simulink model "PRO_TestHarness"  (Simulink 8.6)
settings: Solver=ode45  StartTime=0.0  StopTime=10.0  RelTol=1e-3
PreLoadFcn:
  | addpath('./Workspace/')
  | load('./Workspace/EnvVar.mat')
  | if exist('tl_preloadfcn','file'), tl_preloadfcn(gcs,402); end
PostLoadFcn:
  | if exist('tl_postloadfcn','file'), tl_postloadfcn(gcs,402); end
InitFcn:
  | if exist('tlds_init','file'), tlds_init(gcs); end
StartFcn:
  | if exist('tlds_start','file'), tlds_start(gcs); end
StopFcn:
  | if exist('tlds_stop','file'), tlds_stop(gcs); end
undefined symbols (not defined in the file or in its folder): ddv, sigbuilder_block, Ts
libraries: tllib x19, simulink x2
(part 4 of 5)

== system PRO_TestHarness/PRO_AC_ProductionCycles/Subsystem/PRO_AC_ProductionCycles/PRO_AC_ProductionCycles/PRO_runProductionCycles/PRO enabled/FctCommonPROManageInputs/FctCommonEvaluatePreConditions ==
  b8SystemContextInhibition : Inport  OutDataTypeStr=uint8  PortDimensions=1
  b8SystemContextAbortion : Inport  Port=2  OutDataTypeStr=uint8  PortDimensions=1
  bNoInhibitionByUVDuringTensioning : Inport  Port=3  OutDataTypeStr=boolean
  u8OverVoltageEventStatus : Inport  Port=4
  Bitwise Operator : tllib/Bitwise Operator  logicop=AND  UseBitMask=off  NumInputPorts=2  BitMask=bin2dec('11011001')  BitMaskRealWorld=Stored Integer  data={'date',735742.74357686343}
  Constant2 : Constant  Value=ddv('BFD/KU8_CONTEXT_STATUS_ON')  OutDataTypeStr=uint8  mask(TL_Constant){data={'output',{'variable','BFD/KU8_CONTEXT_STATUS_ON'},'date',735893.58242878469}}
      settings: DeleteFcn=if exist('delete_tlblock','file')==2,delete_tlblock(gcbh);end  NameChangeFcn=if exist('rename_tlblock','file')==2,rename_tlblock(gcbh);end  OpenFcn=if exist('tl_open_blockdlg','file')==2,tl_open_blockdlg(gcbh);else,open_system(gcbh,'parameter');end
      mask Help: eval(['if exist(''tl_online_help'',''file'') == 2, tl_online_help(''Topic'',''TL_Constant''),else, web([''jar:file:///'',matlabroot,''/help/toolbox/simulink/help.jar!/slref/' lower(get_param(gcbh,'Blocktype')) '.html''], ''-helpbrowser''),end'])
      mask Display: plot([-0.05, 1.05, NaN, -0.05, 1.05],[.01, .01, NaN, .99, .99])
  Constant3 : Constant  Value=ddv('BFD/KU8_ZERO')  OutDataTypeStr=uint8  mask(TL_Constant){data={'output',{'variable','BFD/KU8_ZERO'},'date',735742.74390618061}}
      settings: DeleteFcn=if exist('delete_tlblock','file')==2,delete_tlblock(gcbh);end  NameChangeFcn=if exist('rename_tlblock','file')==2,rename_tlblock(gcbh);end  OpenFcn=if exist('tl_open_blockdlg','file')==2,tl_open_blockdlg(gcbh);else,open_system(gcbh,'parameter');end
      mask Help: eval(['if exist(''tl_online_help'',''file'') == 2, tl_online_help(''Topic'',''TL_Constant''),else, web([''jar:file:///'',matlabroot,''/help/toolbox/simulink/help.jar!/slref/' lower(get_param(gcbh,'Blocktype')) '.html''], ''-helpbrowser''),end'])
      mask Display: plot([-0.05, 1.05, NaN, -0.05, 1.05],[.01, .01, NaN, .99, .99])
  Constant4 : Constant  Value=ddv('BFD/KU8_CONTEXT_STATUS_ON')  OutDataTypeStr=uint8  mask(TL_Constant){data={'output',{'variable','BFD/KU8_CONTEXT_STATUS_ON'},'date',735893.58242917829}}
      settings: DeleteFcn=if exist('delete_tlblock','file')==2,delete_tlblock(gcbh);end  NameChangeFcn=if exist('rename_tlblock','file')==2,rename_tlblock(gcbh);end  OpenFcn=if exist('tl_open_blockdlg','file')==2,tl_open_blockdlg(gcbh);else,open_system(gcbh,'parameter');end
      mask Help: eval(['if exist(''tl_online_help'',''file'') == 2, tl_online_help(''Topic'',''TL_Constant''),else, web([''jar:file:///'',matlabroot,''/help/toolbox/simulink/help.jar!/slref/' lower(get_param(gcbh,'Blocktype')) '.html''], ''-helpbrowser''),end'])
      mask Display: plot([-0.05, 1.05, NaN, -0.05, 1.05],[.01, .01, NaN, .99, .99])
  Constant5 : Constant  Value=ddv('RTE_DEFINES/DEM_UDS_STATUS_TF')  OutDataTypeStr=uint8  mask(TL_Constant){data={'output',{'variable','RTE_DEFINES/DEM_UDS_STATUS_TF'},'date',736811.33803680551}}
      settings: DeleteFcn=if exist('delete_tlblock','file')==2,delete_tlblock(gcbh);end  NameChangeFcn=if exist('rename_tlblock','file')==2,rename_tlblock(gcbh);end  OpenFcn=if exist('tl_open_blockdlg','file')==2,tl_open_blockdlg(gcbh);else,open_system(gcbh,'parameter');end
      mask Help: eval(['if exist(''tl_online_help'',''file'') == 2, tl_online_help(''Topic'',''TL_Constant''),else, web([''jar:file:///'',matlabroot,''/help/toolbox/simulink/help.jar!/slref/' lower(get_param(gcbh,'Blocktype')) '.html''], ''-helpbrowser''),end'])
      mask Display: plot([-0.05, 1.05, NaN, -0.05, 1.05],[.01, .01, NaN, .99, .99])
  Function : tllib/Function  data={'stepfunctionname','EvaluatePreConditionsForAllPRO','stepfunctionclass','STATIC_FCN_ASR4','codecomment',['This function is in charge of' char(10) 'providing the following outputs:' char(10) '' char(10) '- the common PRO preconditions flag' char(10) '' char(10) 'according to the inputs:' char(10) '' char(10) '- inhibition context' char(10) '- abortion context'],'module','PRO_AC_ProductionCycles','date',736463.55392600689}  displayString=FUNCTION
  Relational Operator3 : RelationalOperator  Operator=~=  OutDataTypeStr=boolean  mask(TL_RelationalOperator){data={'date',735893.57161760412}}
      settings: DeleteFcn=if exist('delete_tlblock','file')==2,delete_tlblock(gcbh);end  NameChangeFcn=if exist('rename_tlblock','file')==2,rename_tlblock(gcbh);end  OpenFcn=if exist('tl_open_blockdlg','file')==2,tl_open_blockdlg(gcbh);else,open_system(gcbh,'parameter');end
      mask Help: eval(['if exist(''tl_online_help'',''file'') == 2, tl_online_help(''Topic'',''TL_RelationalOperator''),else, web([''jar:file:///'',matlabroot,''/help/toolbox/simulink/help.jar!/slref/' lower(get_param(gcbh,'Blocktype')) '.html''], ''-helpbrowser''),end'])
      mask Display: plot([-0.05, 1.05, NaN, -0.05, 1.05],[.01, .01, NaN, .99, .99])
  Relational Operator4 : RelationalOperator  Operator=~=  OutDataTypeStr=boolean  mask(TL_RelationalOperator){data={'date',735893.57182078704}}
      settings: DeleteFcn=if exist('delete_tlblock','file')==2,delete_tlblock(gcbh);end  NameChangeFcn=if exist('rename_tlblock','file')==2,rename_tlblock(gcbh);end  OpenFcn=if exist('tl_open_blockdlg','file')==2,tl_open_blockdlg(gcbh);else,open_system(gcbh,'parameter');end
      mask Help: eval(['if exist(''tl_online_help'',''file'') == 2, tl_online_help(''Topic'',''TL_RelationalOperator''),else, web([''jar:file:///'',matlabroot,''/help/toolbox/simulink/help.jar!/slref/' lower(get_param(gcbh,'Blocktype')) '.html''], ''-helpbrowser''),end'])
      mask Display: plot([-0.05, 1.05, NaN, -0.05, 1.05],[.01, .01, NaN, .99, .99])
  bOVONotQualified : RelationalOperator  Operator===  OutDataTypeStr=boolean  mask(TL_RelationalOperator){data={'output',{'name','$B'},'date',735987.61379924766}}
      settings: DeleteFcn=if exist('delete_tlblock','file')==2,delete_tlblock(gcbh);end  NameChangeFcn=if exist('rename_tlblock','file')==2,rename_tlblock(gcbh);end  OpenFcn=if exist('tl_open_blockdlg','file')==2,tl_open_blockdlg(gcbh);else,open_system(gcbh,'parameter');end
      mask Help: eval(['if exist(''tl_online_help'',''file'') == 2, tl_online_help(''Topic'',''TL_RelationalOperator''),else, web([''jar:file:///'',matlabroot,''/help/toolbox/simulink/help.jar!/slref/' lower(get_param(gcbh,'Blocktype')) '.html''], ''-helpbrowser''),end'])
      mask Display: plot([-0.05, 1.05, NaN, -0.05, 1.05],[.01, .01, NaN, .99, .99])
  bPreConditionsFlag_PRO : Logic  Inputs=4  AllPortsSameDT=off  OutDataTypeStr=boolean  mask(TL_LogicalOperator){data={'output',{'name','$B'},'date',735986.42247924767}}
      settings: DeleteFcn=if exist('delete_tlblock','file')==2,delete_tlblock(gcbh);end  NameChangeFcn=if exist('rename_tlblock','file')==2,rename_tlblock(gcbh);end  OpenFcn=if exist('tl_open_blockdlg','file')==2,tl_open_blockdlg(gcbh);else,open_system(gcbh,'parameter');end
      mask Help: eval(['if exist(''tl_online_help'',''file'') == 2, tl_online_help(''Topic'',''TL_LogicalOperator''),else, web([''jar:file:///'',matlabroot,''/help/toolbox/simulink/help.jar!/slref/' lower(get_param(gcbh,'Blocktype')) '.html''], ''-helpbrowser''),end'])
      mask Display: plot([-0.05, 1.05, NaN, -0.05, 1.05],[.01, .01, NaN, .99, .99])
  bPreConditionsFlagT_out : Outport  InitialOutput=[0]
  wires:
  b8SystemContextInhibition/1 -> Relational Operator3/1
  Constant2/1 -> Relational Operator3/2
  Constant4/1 -> Relational Operator4/2
  b8SystemContextAbortion/1 -> Relational Operator4/1
  Relational Operator4/1 -> bPreConditionsFlag_PRO/2
  Relational Operator3/1 -> bPreConditionsFlag_PRO/1
  bPreConditionsFlag_PRO/1 -> bPreConditionsFlagT_out/1
  bNoInhibitionByUVDuringTensioning/1 -> bPreConditionsFlag_PRO/3
  bOVONotQualified/1 -> bPreConditionsFlag_PRO/4
  Constant5/1 -> Bitwise Operator/2
  Bitwise Operator/1 -> bOVONotQualified/1
  Constant3/1 -> bOVONotQualified/2
  u8OverVoltageEventStatus/1 -> Bitwise Operator/1

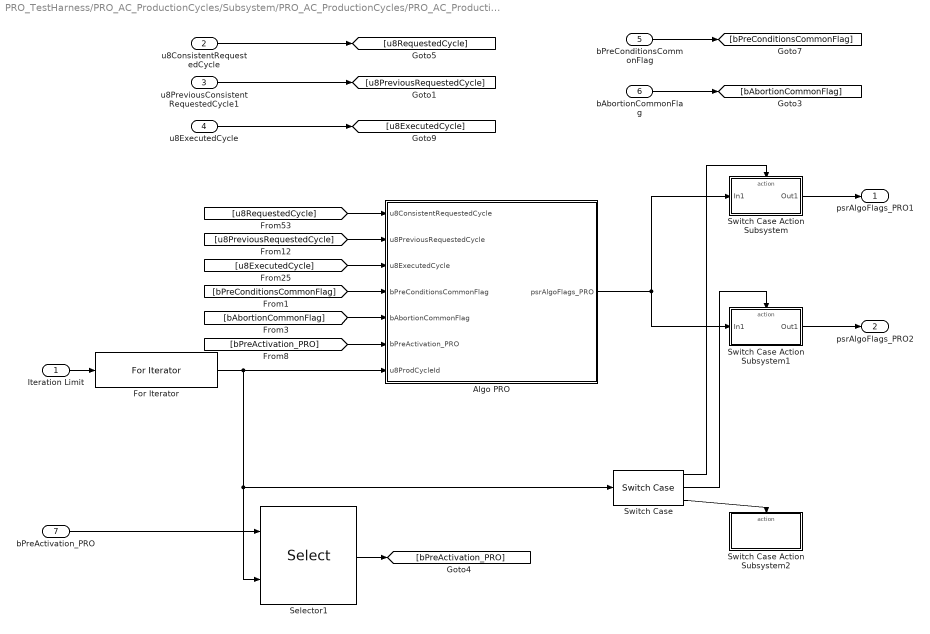
== system PRO_TestHarness/PRO_AC_ProductionCycles/Subsystem/PRO_AC_ProductionCycles/PRO_AC_ProductionCycles/PRO_runProductionCycles/PRO enabled/FctTrigAbortCycle_AllPRO/For Iterator Subsystem ==
  Iteration Limit : Inport
  u8ConsistentRequestedCycle : Inport  Port=2  OutDataTypeStr=uint8  PortDimensions=1
  u8PreviousConsistentRequestedCycle1 : Inport  Port=3  OutDataTypeStr=uint8  PortDimensions=1
  u8ExecutedCycle : Inport  Port=4  PortDimensions=1
  bPreConditionsCommonFlag : Inport  Port=5
  bAbortionCommonFlag : Inport  Port=6  PortDimensions=1
  bPreActivation_PRO : Inport  Port=7
  Algo PRO : Subsystem
  For Iterator : ForIterator  IterationSource=external  IndexMode=Zero-based  IterationVariableDataType=int8
  Selector1 : Selector  IndexMode=Zero-based  InputPortWidth=2  IndexOptions=Index vector (port)  Indices=[1 3]  OutputSizes=1
  Switch Case : SwitchCase  CaseConditions={0,1}
  Switch Case Action Subsystem : Subsystem  TreatAsAtomicUnit=on
  Switch Case Action Subsystem1 : Subsystem  TreatAsAtomicUnit=on
  Switch Case Action Subsystem2 : Subsystem  TreatAsAtomicUnit=on
  psrAlgoFlags_PRO1 : Outport
  psrAlgoFlags_PRO2 : Outport  Port=2
  wires:
  Algo PRO/1(psrAlgoFlags_PRO) -> Switch Case Action Subsystem1/1(In1), Switch Case Action Subsystem/1(In1)
  Iteration Limit/1 -> For Iterator/1
  u8ExecutedCycle/1 -> [u8ExecutedCycle]
  bAbortionCommonFlag/1 -> [bAbortionCommonFlag]
  bPreConditionsCommonFlag/1 -> [bPreConditionsCommonFlag]
  u8ConsistentRequestedCycle/1 -> [u8RequestedCycle]
  bPreActivation_PRO/1 -> Selector1/1
  u8PreviousConsistentRequestedCycle1/1 -> [u8PreviousRequestedCycle]
  For Iterator/1 -> Selector1/2, Switch Case/1, Algo PRO/7(u8ProdCycleId)
  [bPreConditionsCommonFlag] -> Algo PRO/4(bPreConditionsCommonFlag)
  [u8RequestedCycle] -> Algo PRO/1(u8ConsistentRequestedCycle)
  [bPreActivation_PRO] -> Algo PRO/6(bPreActivation_PRO)
  [bAbortionCommonFlag] -> Algo PRO/5(bAbortionCommonFlag)
  [u8PreviousRequestedCycle] -> Algo PRO/2(u8PreviousRequestedCycle)
  [u8ExecutedCycle] -> Algo PRO/3(u8ExecutedCycle)
  Switch Case/1 -> Switch Case Action Subsystem/Action
  Switch Case Action Subsystem/1(Out1) -> psrAlgoFlags_PRO1/1
  Switch Case Action Subsystem1/1(Out1) -> psrAlgoFlags_PRO2/1
  Switch Case/2 -> Switch Case Action Subsystem1/Action
  Switch Case/3 -> Switch Case Action Subsystem2/Action
  Selector1/1 -> [bPreActivation_PRO]

== system PRO_TestHarness/PRO_AC_ProductionCycles/Subsystem/PRO_AC_ProductionCycles/PRO_AC_ProductionCycles/PRO_runProductionCycles/PRO enabled/FctCommonPROManageInputs/FctCheckUnderVoltageDuringTensioningForAllPRO/For Iterator Subsystem ==
  In1 : Inport
  bPreActivationFlag_PRO : Inport  Port=2
  bPreActivationFlag_PRO_UnitDelay : Inport  Port=3
  Constant : Constant  Value=0  OutDataTypeStr=boolean  mask(TL_Constant){data={'date',736182.47245412041}}
      settings: CopyFcn=if exist('tl_reset_reviewflag') == 2, tl_reset_reviewflag(gcbh); end  DeleteFcn=if exist('delete_tlblock','file')==2,delete_tlblock(gcbh);end  NameChangeFcn=if exist('rename_tlblock','file')==2,rename_tlblock(gcbh);end  OpenFcn=if exist('tl_open_blockdlg','file')==2,tl_open_blockdlg(gcbh);else,open_system(gcbh,'parameter');end
      mask Help: eval(['if exist(''tl_online_help'',''file'') == 2, tl_online_help(''Topic'',''TL_Constant''),else, web([''jar:file:///'',matlabroot,''/help/toolbox/simulink/help.jar!/slref/' lower(get_param(gcbh,'Blocktype')) '.html''], ''-helpbrowser''),end'])
      mask Display: plot([-0.05, 1.05, NaN, -0.05, 1.05],[.01, .01, NaN, .99, .99])
  For Iterator : ForIterator  IterationSource=external  IndexMode=Zero-based  IterationVariableDataType=int8
  Selector : Selector  IndexMode=Zero-based  InputPortWidth=2  IndexOptions=Index vector (port)  Indices=[1 3]  OutputSizes=1
  Selector1 : Selector  IndexMode=Zero-based  InputPortWidth=2  IndexOptions=Index vector (port)  Indices=[1 3]  OutputSizes=1
  Switch : Switch  Criteria=u2 ~= 0  mask(TL_Switch){data={'output',{'type','Bool'},'date',736182.47204471065}}
      settings: CopyFcn=if exist('tl_reset_reviewflag') == 2, tl_reset_reviewflag(gcbh); end  DeleteFcn=if exist('delete_tlblock','file')==2,delete_tlblock(gcbh);end  NameChangeFcn=if exist('rename_tlblock','file')==2,rename_tlblock(gcbh);end  OpenFcn=if exist('tl_open_blockdlg','file')==2,tl_open_blockdlg(gcbh);else,open_system(gcbh,'parameter');end
      mask Help: eval(['if exist(''tl_online_help'',''file'') == 2, tl_online_help(''Topic'',''TL_Switch''),else, web([''jar:file:///'',matlabroot,''/help/toolbox/simulink/help.jar!/slref/' lower(get_param(gcbh,'Blocktype')) '.html''], ''-helpbrowser''),end'])
      mask Display: plot([-0.05, 1.05, NaN, -0.05, 1.05],[.01, .01, NaN, .99, .99])
  Unit Delay : UnitDelay  SampleTime=-1  mask(TL_UnitDelay){data={'output',{'type','Bool'},'state',{'name','X_bIterationMemory','type','Bool'},'date',736182.47589184029}}
      settings: CopyFcn=if exist('tl_reset_reviewflag') == 2, tl_reset_reviewflag(gcbh); end  DeleteFcn=if exist('delete_tlblock','file')==2,delete_tlblock(gcbh);end  NameChangeFcn=if exist('rename_tlblock','file')==2,rename_tlblock(gcbh);end  OpenFcn=if exist('tl_open_blockdlg','file')==2,tl_open_blockdlg(gcbh);else,open_system(gcbh,'parameter');end
      mask Help: eval(['if exist(''tl_online_help'',''file'') == 2, tl_online_help(''Topic'',''TL_UnitDelay''),else, web([''jar:file:///'',matlabroot,''/help/toolbox/simulink/help.jar!/slref/' lower(get_param(gcbh,'Blocktype')) '.html''], ''-helpbrowser''),end'])
      mask Display: plot([-0.05, 1.05, NaN, -0.05, 1.05],[.01, .01, NaN, .99, .99])
  bNewRequest : Logic  AllPortsSameDT=off  OutDataTypeStr=boolean  mask(TL_LogicalOperator){data={'output',{'name','$B'},'date',735907.68610908568}}
      settings: DeleteFcn=if exist('delete_tlblock','file')==2,delete_tlblock(gcbh);end  NameChangeFcn=if exist('rename_tlblock','file')==2,rename_tlblock(gcbh);end  OpenFcn=if exist('tl_open_blockdlg','file')==2,tl_open_blockdlg(gcbh);else,open_system(gcbh,'parameter');end
      mask Help: eval(['if exist(''tl_online_help'',''file'') == 2, tl_online_help(''Topic'',''TL_LogicalOperator''),else, web([''jar:file:///'',matlabroot,''/help/toolbox/simulink/help.jar!/slref/' lower(get_param(gcbh,'Blocktype')) '.html''], ''-helpbrowser''),end'])
      mask Display: plot([-0.05, 1.05, NaN, -0.05, 1.05],[.01, .01, NaN, .99, .99])
  bNewRequest_PRO : Logic  Operator=OR  AllPortsSameDT=off  OutDataTypeStr=boolean  mask(TL_LogicalOperator){data={'output',{'name','$B'},'date',736182.47130738432}}
      settings: DeleteFcn=if exist('delete_tlblock','file')==2,delete_tlblock(gcbh);end  NameChangeFcn=if exist('rename_tlblock','file')==2,rename_tlblock(gcbh);end  OpenFcn=if exist('tl_open_blockdlg','file')==2,tl_open_blockdlg(gcbh);else,open_system(gcbh,'parameter');end
      mask Help: eval(['if exist(''tl_online_help'',''file'') == 2, tl_online_help(''Topic'',''TL_LogicalOperator''),else, web([''jar:file:///'',matlabroot,''/help/toolbox/simulink/help.jar!/slref/' lower(get_param(gcbh,'Blocktype')) '.html''], ''-helpbrowser''),end'])
      mask Display: plot([-0.05, 1.05, NaN, -0.05, 1.05],[.01, .01, NaN, .99, .99])
  bNoPreviousPreActivation_PRO : Logic  Operator=NOT  Inputs=1  AllPortsSameDT=off  OutDataTypeStr=boolean  mask(TL_LogicalOperator){data={'output',{'name','$B'},'date',735910.63061995374}}
      settings: DeleteFcn=if exist('delete_tlblock','file')==2,delete_tlblock(gcbh);end  NameChangeFcn=if exist('rename_tlblock','file')==2,rename_tlblock(gcbh);end  OpenFcn=if exist('tl_open_blockdlg','file')==2,tl_open_blockdlg(gcbh);else,open_system(gcbh,'parameter');end
      mask Help: eval(['if exist(''tl_online_help'',''file'') == 2, tl_online_help(''Topic'',''TL_LogicalOperator''),else, web([''jar:file:///'',matlabroot,''/help/toolbox/simulink/help.jar!/slref/' lower(get_param(gcbh,'Blocktype')) '.html''], ''-helpbrowser''),end'])
      mask Display: plot([-0.05, 1.05, NaN, -0.05, 1.05],[.01, .01, NaN, .99, .99])
  Out1 : Outport
  wires:
  Selector/1 -> bNewRequest/1
  bNoPreviousPreActivation_PRO/1 -> bNewRequest/2
  Selector1/1 -> bNoPreviousPreActivation_PRO/1
  bNewRequest/1 -> bNewRequest_PRO/1
  In1/1 -> For Iterator/1
  bPreActivationFlag_PRO/1 -> Selector/1
  For Iterator/1 -> Selector1/2, Switch/2, Selector/2
  bNewRequest_PRO/1 -> Unit Delay/1, Out1/1
  Switch/1 -> bNewRequest_PRO/2
  Constant/1 -> Switch/3
  Unit Delay/1 -> Switch/1
  bPreActivationFlag_PRO_UnitDelay/1 -> Selector1/1

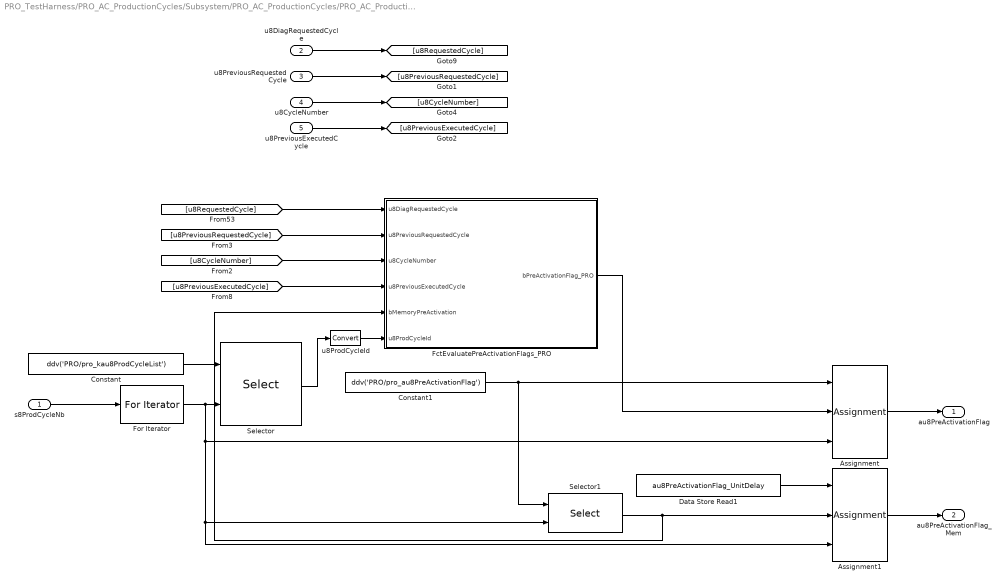
== system PRO_TestHarness/PRO_AC_ProductionCycles/Subsystem/PRO_AC_ProductionCycles/PRO_AC_ProductionCycles/PRO_runProductionCycles/PRO enabled/FctCommonPROManageInputs/FctCommonEvaluatePreActivationFlags/For Iterator Subsystem ==
  s8ProdCycleNb : Inport
  u8DiagRequestedCycle : Inport  Port=2  OutDataTypeStr=uint8  PortDimensions=1
  u8PreviousRequestedCycle : Inport  Port=3  OutDataTypeStr=uint8  PortDimensions=1
  u8CycleNumber : Inport  Port=4  PortDimensions=1
  u8PreviousExecutedCycle : Inport  Port=5  PortDimensions=1
  Assignment : Assignment  IndexMode=Zero-based  IndexOptions=Index vector (port)  Indices=1  OutputSizes=1  mask(TL_Assignment){data={'output',{'variable','PRO/pro_au8PreActivationFlag','inheritscaling',0},'date',736182.43548592587}}
      settings: CopyFcn=if exist('tl_reset_reviewflag') == 2, tl_reset_reviewflag(gcbh); end  DeleteFcn=if exist('delete_tlblock','file')==2,delete_tlblock(gcbh);end  NameChangeFcn=if exist('rename_tlblock','file')==2,rename_tlblock(gcbh);end  OpenFcn=if exist('tl_open_blockdlg','file')==2,tl_open_blockdlg(gcbh);else,open_system(gcbh,'parameter');end
      mask Help: eval(['if exist(''tl_online_help'',''file'') == 2, tl_online_help(''Topic'',''TL_Assignment''),else, web([''jar:file:///'',matlabroot,''/help/toolbox/simulink/help.jar!/slref/' lower(get_param(gcbh,'Blocktype')) '.html''], ''-helpbrowser''),end'])
      mask Display: plot([-0.05, 1.05, NaN, -0.05, 1.05],[.01, .01, NaN, .99, .99])
  Assignment1 : Assignment  IndexMode=Zero-based  IndexOptions=Index vector (port)  Indices=1  OutputSizes=1  mask(TL_Assignment){data={'output',{'variable','PRO/pro_au8PreActivationFlag_UnitDelay','inheritscaling',0},'date',736182.54364810186}}
      settings: CopyFcn=if exist('tl_reset_reviewflag') == 2, tl_reset_reviewflag(gcbh); end  DeleteFcn=if exist('delete_tlblock','file')==2,delete_tlblock(gcbh);end  NameChangeFcn=if exist('rename_tlblock','file')==2,rename_tlblock(gcbh);end  OpenFcn=if exist('tl_open_blockdlg','file')==2,tl_open_blockdlg(gcbh);else,open_system(gcbh,'parameter');end
      mask Help: eval(['if exist(''tl_online_help'',''file'') == 2, tl_online_help(''Topic'',''TL_Assignment''),else, web([''jar:file:///'',matlabroot,''/help/toolbox/simulink/help.jar!/slref/' lower(get_param(gcbh,'Blocktype')) '.html''], ''-helpbrowser''),end'])
      mask Display: plot([-0.05, 1.05, NaN, -0.05, 1.05],[.01, .01, NaN, .99, .99])
  Constant : Constant  Value=ddv('PRO/pro_kau8ProdCycleList')  mask(TL_Constant){data={'output',{'variable','PRO/pro_kau8ProdCycleList'},'date',736182.43287164357}}
      settings: CopyFcn=if exist('tl_reset_reviewflag') == 2, tl_reset_reviewflag(gcbh); end  DeleteFcn=if exist('delete_tlblock','file')==2,delete_tlblock(gcbh);end  NameChangeFcn=if exist('rename_tlblock','file')==2,rename_tlblock(gcbh);end  OpenFcn=if exist('tl_open_blockdlg','file')==2,tl_open_blockdlg(gcbh);else,open_system(gcbh,'parameter');end
      mask Help: eval(['if exist(''tl_online_help'',''file'') == 2, tl_online_help(''Topic'',''TL_Constant''),else, web([''jar:file:///'',matlabroot,''/help/toolbox/simulink/help.jar!/slref/' lower(get_param(gcbh,'Blocktype')) '.html''], ''-helpbrowser''),end'])
      mask Display: plot([-0.05, 1.05, NaN, -0.05, 1.05],[.01, .01, NaN, .99, .99])
  Constant1 : Constant  Value=ddv('PRO/pro_au8PreActivationFlag')  OutDataTypeStr=boolean  mask(TL_Constant){data={'output',{'variable','PRO/pro_au8PreActivationFlag'},'date',736183.46763438662}}
      settings: CopyFcn=if exist('tl_reset_reviewflag') == 2, tl_reset_reviewflag(gcbh); end  DeleteFcn=if exist('delete_tlblock','file')==2,delete_tlblock(gcbh);end  NameChangeFcn=if exist('rename_tlblock','file')==2,rename_tlblock(gcbh);end  OpenFcn=if exist('tl_open_blockdlg','file')==2,tl_open_blockdlg(gcbh);else,open_system(gcbh,'parameter');end
      mask Help: eval(['if exist(''tl_online_help'',''file'') == 2, tl_online_help(''Topic'',''TL_Constant''),else, web([''jar:file:///'',matlabroot,''/help/toolbox/simulink/help.jar!/slref/' lower(get_param(gcbh,'Blocktype')) '.html''], ''-helpbrowser''),end'])
      mask Display: plot([-0.05, 1.05, NaN, -0.05, 1.05],[.01, .01, NaN, .99, .99])
  Data Store Read1 : DataStoreRead  DataStoreName=au8PreActivationFlag_UnitDelay  mask(TL_DataStoreRead){data={'date',736183.33570861106}}
      settings: DeleteFcn=if exist('delete_tlblock','file')==2,delete_tlblock(gcbh);end  NameChangeFcn=if exist('rename_tlblock','file')==2,rename_tlblock(gcbh);end  OpenFcn=if exist('tl_open_blockdlg','file')==2,tl_open_blockdlg(gcbh);else,open_system(gcbh,'parameter');end
      mask Help: eval(['if exist(''tl_online_help'',''file'') == 2, tl_online_help(''Topic'',''TL_DataStoreRead''),else, web([''jar:file:///'',matlabroot,''/help/toolbox/simulink/help.jar!/slref/' lower(get_param(gcbh,'Blocktype')) '.html''], ''-helpbrowser''),end'])
      mask Display: plot([-0.05, 1.05, NaN, -0.05, 1.05],[.01, .01, NaN, .99, .99])
  FctEvaluatePreActivationFlags_PRO : Subsystem  TreatAsAtomicUnit=on
  For Iterator : ForIterator  IterationSource=external  IndexMode=Zero-based  IterationVariableDataType=int8
  Selector : Selector  IndexMode=Zero-based  InputPortWidth=2  IndexOptions=Index vector (port)  Indices=[1 3]  OutputSizes=1
  Selector1 : Selector  IndexMode=Zero-based  InputPortWidth=2  IndexOptions=Index vector (port)  Indices=[1 3]  OutputSizes=1
  u8ProdCycleId : DataTypeConversion  mask(TL_Rescaler){data={'output',{'name','$B','type','UInt8'},'date',736169.63813659723}}
      settings: DeleteFcn=if exist('delete_tlblock','file')==2,delete_tlblock(gcbh);end  NameChangeFcn=if exist('rename_tlblock','file')==2,rename_tlblock(gcbh);end  OpenFcn=if exist('tl_open_blockdlg','file')==2,tl_open_blockdlg(gcbh);else,open_system(gcbh,'parameter');end
      mask Help: eval(['if exist(''tl_online_help'',''file'') == 2, tl_online_help(''Topic'',''TL_Rescaler''),else, web([''jar:file:///'',matlabroot,''/help/toolbox/simulink/help.jar!/slref/' lower(get_param(gcbh,'Blocktype')) '.html''], ''-helpbrowser''),end'])
      mask Display: plot([-0.05, 1.05, NaN, -0.05, 1.05],[.01, .01, NaN, .99, .99])
  au8PreActivationFlag : Outport
  au8PreActivationFlag_Mem : Outport  Port=2
  wires:
  u8CycleNumber/1 -> [u8CycleNumber]
  u8DiagRequestedCycle/1 -> [u8RequestedCycle]
  u8PreviousExecutedCycle/1 -> [u8PreviousExecutedCycle]
  u8PreviousRequestedCycle/1 -> [u8PreviousRequestedCycle]
  [u8PreviousRequestedCycle] -> FctEvaluatePreActivationFlags_PRO/2(u8PreviousRequestedCycle)
  [u8PreviousExecutedCycle] -> FctEvaluatePreActivationFlags_PRO/4(u8PreviousExecutedCycle)
  [u8RequestedCycle] -> FctEvaluatePreActivationFlags_PRO/1(u8DiagRequestedCycle)
  [u8CycleNumber] -> FctEvaluatePreActivationFlags_PRO/3(u8CycleNumber)
  u8ProdCycleId/1 -> FctEvaluatePreActivationFlags_PRO/6(u8ProdCycleId)
  For Iterator/1 -> Selector1/2, Assignment1/3, Assignment/3, Selector/2
  Selector/1 -> u8ProdCycleId/1
  Constant/1 -> Selector/1
  s8ProdCycleNb/1 -> For Iterator/1
  Assignment/1 -> au8PreActivationFlag/1
  Constant1/1 -> Selector1/1, Assignment/1
  FctEvaluatePreActivationFlags_PRO/1(bPreActivationFlag_PRO) -> Assignment/2
  Assignment1/1 -> au8PreActivationFlag_Mem/1
  Data Store Read1/1 -> Assignment1/1
  Selector1/1 -> Assignment1/2, FctEvaluatePreActivationFlags_PRO/5(bMemoryPreActivation)

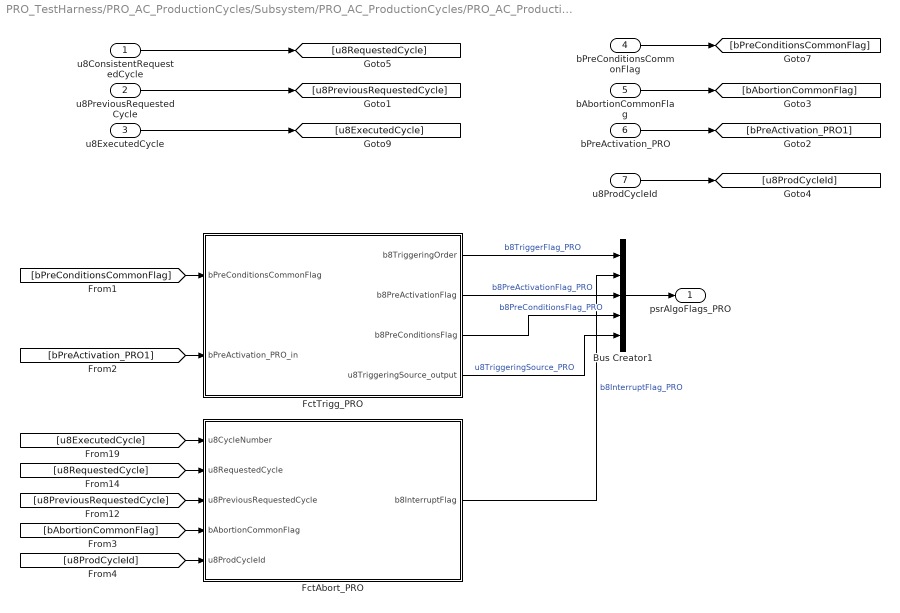
== system PRO_TestHarness/PRO_AC_ProductionCycles/Subsystem/PRO_AC_ProductionCycles/PRO_AC_ProductionCycles/PRO_runProductionCycles/PRO enabled/FctTrigAbortCycle_AllPRO/For Iterator Subsystem/Algo PRO ==
  u8ConsistentRequestedCycle : Inport  OutDataTypeStr=uint8  PortDimensions=1
  u8PreviousRequestedCycle : Inport  Port=2  OutDataTypeStr=uint8  PortDimensions=1
  u8ExecutedCycle : Inport  Port=3  PortDimensions=1
  bPreConditionsCommonFlag : Inport  Port=4
  bAbortionCommonFlag : Inport  Port=5  PortDimensions=1
  bPreActivation_PRO : Inport  Port=6
  u8ProdCycleId : Inport  Port=7  PortDimensions=1
  Bus Creator1 : BusCreator  Inputs=5
  FctAbort_PRO : Subsystem  TreatAsAtomicUnit=on
  FctTrigg_PRO : Subsystem  TreatAsAtomicUnit=on
  psrAlgoFlags_PRO : Outport
  wires:
  [u8ExecutedCycle] -> FctAbort_PRO/1(u8CycleNumber)
  [u8RequestedCycle] -> FctAbort_PRO/2(u8RequestedCycle)
  [bAbortionCommonFlag] -> FctAbort_PRO/4(bAbortionCommonFlag)
  Bus Creator1/1 -> psrAlgoFlags_PRO/1
  FctTrigg_PRO/1(b8TriggeringOrder) -> Bus Creator1/1  "b8TriggerFlag_PRO"
  FctTrigg_PRO/4(u8TriggeringSource_output) -> Bus Creator1/5  "u8TriggeringSource_PRO"
  FctTrigg_PRO/2(b8PreActivationFlag) -> Bus Creator1/3  "b8PreActivationFlag_PRO"
  FctTrigg_PRO/3(b8PreConditionsFlag) -> Bus Creator1/4  "b8PreConditionsFlag_PRO"
  FctAbort_PRO/1(b8InterruptFlag) -> Bus Creator1/2  "b8InterruptFlag_PRO"
  [u8PreviousRequestedCycle] -> FctAbort_PRO/3(u8PreviousRequestedCycle)
  u8ExecutedCycle/1 -> [u8ExecutedCycle]
  bAbortionCommonFlag/1 -> [bAbortionCommonFlag]
  bPreConditionsCommonFlag/1 -> [bPreConditionsCommonFlag]
  u8PreviousRequestedCycle/1 -> [u8PreviousRequestedCycle]
  u8ConsistentRequestedCycle/1 -> [u8RequestedCycle]
  [bPreActivation_PRO1] -> FctTrigg_PRO/2(bPreActivation_PRO_in)
  [bPreConditionsCommonFlag] -> FctTrigg_PRO/1(bPreConditionsCommonFlag)
  bPreActivation_PRO/1 -> [bPreActivation_PRO1]
  u8ProdCycleId/1 -> [u8ProdCycleId]
  [u8ProdCycleId] -> FctAbort_PRO/5(u8ProdCycleId)

== system PRO_TestHarness/PRO_AC_ProductionCycles/Subsystem/PRO_AC_ProductionCycles/PRO_AC_ProductionCycles/PRO_runProductionCycles/PRO enabled/FctTrigAbortCycle_AllPRO/For Iterator Subsystem/Switch Case Action Subsystem ==
  In1 : Inport
  Action Port : ActionPort  ActionType=case
  Out1 : Outport
  wires:
  In1/1 -> Out1/1

== system PRO_TestHarness/PRO_AC_ProductionCycles/Subsystem/PRO_AC_ProductionCycles/PRO_AC_ProductionCycles/PRO_runProductionCycles/PRO enabled/FctTrigAbortCycle_AllPRO/For Iterator Subsystem/Switch Case Action Subsystem1 ==
  In1 : Inport
  Action Port : ActionPort  ActionType=case
  Out1 : Outport
  wires:
  In1/1 -> Out1/1

== system PRO_TestHarness/PRO_AC_ProductionCycles/Subsystem/PRO_AC_ProductionCycles/PRO_AC_ProductionCycles/PRO_runProductionCycles/PRO enabled/FctTrigAbortCycle_AllPRO/For Iterator Subsystem/Switch Case Action Subsystem2 ==
  Action Port : ActionPort  ActionType=default

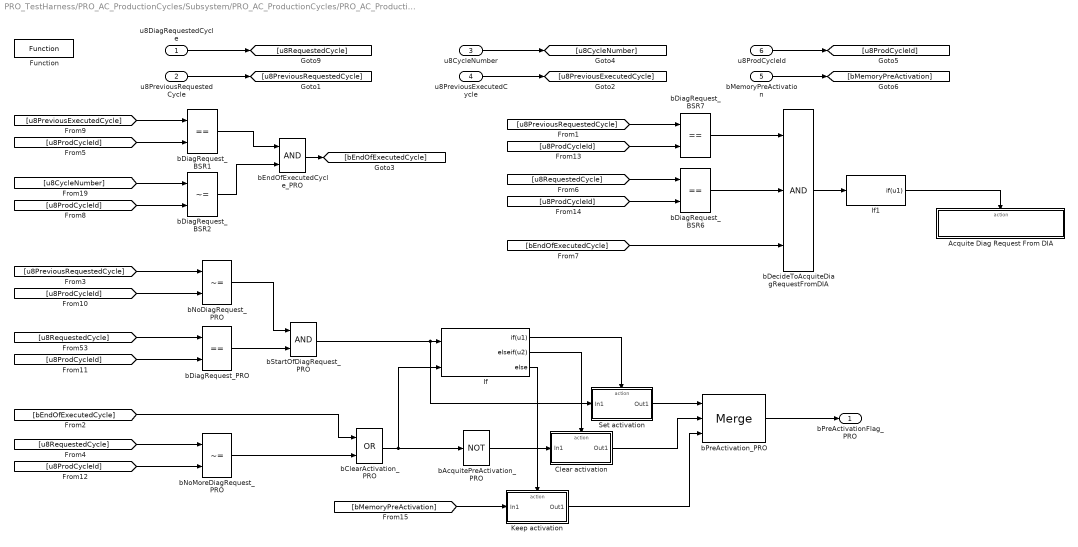
== system PRO_TestHarness/PRO_AC_ProductionCycles/Subsystem/PRO_AC_ProductionCycles/PRO_AC_ProductionCycles/PRO_runProductionCycles/PRO enabled/FctCommonPROManageInputs/FctCommonEvaluatePreActivationFlags/For Iterator Subsystem/FctEvaluatePreActivationFlags_PRO ==
  u8DiagRequestedCycle : Inport  OutDataTypeStr=uint8  PortDimensions=1
  u8PreviousRequestedCycle : Inport  Port=2  OutDataTypeStr=uint8  PortDimensions=1
  u8CycleNumber : Inport  Port=3  PortDimensions=1
  u8PreviousExecutedCycle : Inport  Port=4  PortDimensions=1
  bMemoryPreActivation : Inport  Port=5  PortDimensions=1
  u8ProdCycleId : Inport  Port=6  PortDimensions=1
  Acquite Diag Request From DIA : Subsystem  TreatAsAtomicUnit=on
  Clear activation : Subsystem  TreatAsAtomicUnit=on
  Function : tllib/Function  data={'stepfunctionname','EvaluatePreActivationFlag_PRO','stepfunctionclass','STATIC_FCN_ASR4','codecomment',['This function is in charge of' char(10) 'providing the following outputs:' char(10) '' char(10) '- the common PRO abortion flag' char(10) '' char(10) 'according to the inputs:' char(10) '' char(10) '- abortion context'],'module','PRO_AC_ProductionCycles','date',736463.55391369213}  displayString=FUNCTION
  If : If  NumInputs=2  IfExpression=u1  ElseIfExpressions=u2
  If1 : If  IfExpression=u1  ShowElse=off
  Keep activation : Subsystem  TreatAsAtomicUnit=on
  Set activation : Subsystem  TreatAsAtomicUnit=on
  bAcquitePreActivation_PRO : Logic  Operator=NOT  Inputs=1  AllPortsSameDT=off  OutDataTypeStr=boolean  mask(TL_LogicalOperator){data={'output',{'name','$B'},'date',735791.39028081018}}
      settings: DeleteFcn=if exist('delete_tlblock','file')==2,delete_tlblock(gcbh);end  NameChangeFcn=if exist('rename_tlblock','file')==2,rename_tlblock(gcbh);end  OpenFcn=if exist('tl_open_blockdlg','file')==2,tl_open_blockdlg(gcbh);else,open_system(gcbh,'parameter');end
      mask Help: eval(['if exist(''tl_online_help'',''file'') == 2, tl_online_help(''Topic'',''TL_LogicalOperator''),else, web([''jar:file:///'',matlabroot,''/help/toolbox/simulink/help.jar!/slref/' lower(get_param(gcbh,'Blocktype')) '.html''], ''-helpbrowser''),end'])
      mask Display: plot([-0.05, 1.05, NaN, -0.05, 1.05],[.01, .01, NaN, .99, .99])
  bClearActivation_PRO : Logic  Operator=OR  AllPortsSameDT=off  OutDataTypeStr=boolean  mask(TL_LogicalOperator){data={'output',{'name','$B'},'date',735791.60080171295}}
      settings: DeleteFcn=if exist('delete_tlblock','file')==2,delete_tlblock(gcbh);end  NameChangeFcn=if exist('rename_tlblock','file')==2,rename_tlblock(gcbh);end  OpenFcn=if exist('tl_open_blockdlg','file')==2,tl_open_blockdlg(gcbh);else,open_system(gcbh,'parameter');end
      mask Help: eval(['if exist(''tl_online_help'',''file'') == 2, tl_online_help(''Topic'',''TL_LogicalOperator''),else, web([''jar:file:///'',matlabroot,''/help/toolbox/simulink/help.jar!/slref/' lower(get_param(gcbh,'Blocktype')) '.html''], ''-helpbrowser''),end'])
      mask Display: plot([-0.05, 1.05, NaN, -0.05, 1.05],[.01, .01, NaN, .99, .99])
  bDecideToAcquiteDiagRequestFromDIA : Logic  Inputs=3  AllPortsSameDT=off  OutDataTypeStr=boolean  mask(TL_LogicalOperator){data={'output',{'name','$B'},'date',736039.66169754625}}
      settings: DeleteFcn=if exist('delete_tlblock','file')==2,delete_tlblock(gcbh);end  NameChangeFcn=if exist('rename_tlblock','file')==2,rename_tlblock(gcbh);end  OpenFcn=if exist('tl_open_blockdlg','file')==2,tl_open_blockdlg(gcbh);else,open_system(gcbh,'parameter');end
      mask Help: eval(['if exist(''tl_online_help'',''file'') == 2, tl_online_help(''Topic'',''TL_LogicalOperator''),else, web([''jar:file:///'',matlabroot,''/help/toolbox/simulink/help.jar!/slref/' lower(get_param(gcbh,'Blocktype')) '.html''], ''-helpbrowser''),end'])
      mask Display: plot([-0.05, 1.05, NaN, -0.05, 1.05],[.01, .01, NaN, .99, .99])
  bDiagRequest_BSR1 : RelationalOperator  Operator===  OutDataTypeStr=boolean  mask(TL_RelationalOperator){data={'output',{'name','$B'},'date',735626.40456666669}}
      settings: DeleteFcn=if exist('delete_tlblock','file')==2,delete_tlblock(gcbh);end  NameChangeFcn=if exist('rename_tlblock','file')==2,rename_tlblock(gcbh);end  OpenFcn=if exist('tl_open_blockdlg','file')==2,tl_open_blockdlg(gcbh);else,open_system(gcbh,'parameter');end
      mask Help: eval(['if exist(''tl_online_help'',''file'') == 2, tl_online_help(''Topic'',''TL_RelationalOperator''),else, web([''jar:file:///'',matlabroot,''/help/toolbox/simulink/help.jar!/slref/' lower(get_param(gcbh,'Blocktype')) '.html''], ''-helpbrowser''),end'])
      mask Display: plot([-0.05, 1.05, NaN, -0.05, 1.05],[.01, .01, NaN, .99, .99])
  bDiagRequest_BSR2 : RelationalOperator  Operator=~=  OutDataTypeStr=boolean  mask(TL_RelationalOperator){data={'output',{'name','$B'},'date',736007.62927152775}}
      settings: DeleteFcn=if exist('delete_tlblock','file')==2,delete_tlblock(gcbh);end  NameChangeFcn=if exist('rename_tlblock','file')==2,rename_tlblock(gcbh);end  OpenFcn=if exist('tl_open_blockdlg','file')==2,tl_open_blockdlg(gcbh);else,open_system(gcbh,'parameter');end
      mask Help: eval(['if exist(''tl_online_help'',''file'') == 2, tl_online_help(''Topic'',''TL_RelationalOperator''),else, web([''jar:file:///'',matlabroot,''/help/toolbox/simulink/help.jar!/slref/' lower(get_param(gcbh,'Blocktype')) '.html''], ''-helpbrowser''),end'])
      mask Display: plot([-0.05, 1.05, NaN, -0.05, 1.05],[.01, .01, NaN, .99, .99])
  bDiagRequest_BSR6 : RelationalOperator  Operator===  OutDataTypeStr=boolean  mask(TL_RelationalOperator){data={'output',{'name','$B'},'date',735626.40456666669}}
      settings: DeleteFcn=if exist('delete_tlblock','file')==2,delete_tlblock(gcbh);end  NameChangeFcn=if exist('rename_tlblock','file')==2,rename_tlblock(gcbh);end  OpenFcn=if exist('tl_open_blockdlg','file')==2,tl_open_blockdlg(gcbh);else,open_system(gcbh,'parameter');end
      mask Help: eval(['if exist(''tl_online_help'',''file'') == 2, tl_online_help(''Topic'',''TL_RelationalOperator''),else, web([''jar:file:///'',matlabroot,''/help/toolbox/simulink/help.jar!/slref/' lower(get_param(gcbh,'Blocktype')) '.html''], ''-helpbrowser''),end'])
      mask Display: plot([-0.05, 1.05, NaN, -0.05, 1.05],[.01, .01, NaN, .99, .99])
  bDiagRequest_BSR7 : RelationalOperator  Operator===  OutDataTypeStr=boolean  mask(TL_RelationalOperator){data={'output',{'name','$B'},'date',736039.659091493}}
      settings: DeleteFcn=if exist('delete_tlblock','file')==2,delete_tlblock(gcbh);end  NameChangeFcn=if exist('rename_tlblock','file')==2,rename_tlblock(gcbh);end  OpenFcn=if exist('tl_open_blockdlg','file')==2,tl_open_blockdlg(gcbh);else,open_system(gcbh,'parameter');end
      mask Help: eval(['if exist(''tl_online_help'',''file'') == 2, tl_online_help(''Topic'',''TL_RelationalOperator''),else, web([''jar:file:///'',matlabroot,''/help/toolbox/simulink/help.jar!/slref/' lower(get_param(gcbh,'Blocktype')) '.html''], ''-helpbrowser''),end'])
      mask Display: plot([-0.05, 1.05, NaN, -0.05, 1.05],[.01, .01, NaN, .99, .99])
  bDiagRequest_PRO : RelationalOperator  Operator===  OutDataTypeStr=boolean  mask(TL_RelationalOperator){data={'output',{'name','$B'},'date',735626.40456666669}}
      settings: DeleteFcn=if exist('delete_tlblock','file')==2,delete_tlblock(gcbh);end  NameChangeFcn=if exist('rename_tlblock','file')==2,rename_tlblock(gcbh);end  OpenFcn=if exist('tl_open_blockdlg','file')==2,tl_open_blockdlg(gcbh);else,open_system(gcbh,'parameter');end
      mask Help: eval(['if exist(''tl_online_help'',''file'') == 2, tl_online_help(''Topic'',''TL_RelationalOperator''),else, web([''jar:file:///'',matlabroot,''/help/toolbox/simulink/help.jar!/slref/' lower(get_param(gcbh,'Blocktype')) '.html''], ''-helpbrowser''),end'])
      mask Display: plot([-0.05, 1.05, NaN, -0.05, 1.05],[.01, .01, NaN, .99, .99])
  bEndOfExecutedCycle_PRO : Logic  AllPortsSameDT=off  OutDataTypeStr=boolean  mask(TL_LogicalOperator){data={'output',{'name','$B'},'date',735626.4046887384}}
      settings: DeleteFcn=if exist('delete_tlblock','file')==2,delete_tlblock(gcbh);end  NameChangeFcn=if exist('rename_tlblock','file')==2,rename_tlblock(gcbh);end  OpenFcn=if exist('tl_open_blockdlg','file')==2,tl_open_blockdlg(gcbh);else,open_system(gcbh,'parameter');end
      mask Help: eval(['if exist(''tl_online_help'',''file'') == 2, tl_online_help(''Topic'',''TL_LogicalOperator''),else, web([''jar:file:///'',matlabroot,''/help/toolbox/simulink/help.jar!/slref/' lower(get_param(gcbh,'Blocktype')) '.html''], ''-helpbrowser''),end'])
      mask Display: plot([-0.05, 1.05, NaN, -0.05, 1.05],[.01, .01, NaN, .99, .99])
  bNoDiagRequest_PRO : RelationalOperator  Operator=~=  OutDataTypeStr=boolean  mask(TL_RelationalOperator){data={'output',{'name','$B'},'date',736040.51689770829}}
      settings: DeleteFcn=if exist('delete_tlblock','file')==2,delete_tlblock(gcbh);end  NameChangeFcn=if exist('rename_tlblock','file')==2,rename_tlblock(gcbh);end  OpenFcn=if exist('tl_open_blockdlg','file')==2,tl_open_blockdlg(gcbh);else,open_system(gcbh,'parameter');end
      mask Help: eval(['if exist(''tl_online_help'',''file'') == 2, tl_online_help(''Topic'',''TL_RelationalOperator''),else, web([''jar:file:///'',matlabroot,''/help/toolbox/simulink/help.jar!/slref/' lower(get_param(gcbh,'Blocktype')) '.html''], ''-helpbrowser''),end'])
      mask Display: plot([-0.05, 1.05, NaN, -0.05, 1.05],[.01, .01, NaN, .99, .99])
  bNoMoreDiagRequest_PRO : RelationalOperator  Operator=~=  OutDataTypeStr=boolean  mask(TL_RelationalOperator){data={'output',{'name','$B'},'date',735791.60152292822}}
      settings: DeleteFcn=if exist('delete_tlblock','file')==2,delete_tlblock(gcbh);end  NameChangeFcn=if exist('rename_tlblock','file')==2,rename_tlblock(gcbh);end  OpenFcn=if exist('tl_open_blockdlg','file')==2,tl_open_blockdlg(gcbh);else,open_system(gcbh,'parameter');end
      mask Help: eval(['if exist(''tl_online_help'',''file'') == 2, tl_online_help(''Topic'',''TL_RelationalOperator''),else, web([''jar:file:///'',matlabroot,''/help/toolbox/simulink/help.jar!/slref/' lower(get_param(gcbh,'Blocktype')) '.html''], ''-helpbrowser''),end'])
      mask Display: plot([-0.05, 1.05, NaN, -0.05, 1.05],[.01, .01, NaN, .99, .99])
  bPreActivation_PRO : Merge  Inputs=3  mask(TL_Merge){data={'output',{'name','$B'},'date',735791.38941256946}}
      settings: CopyFcn=if exist('tl_reset_reviewflag') == 2, tl_reset_reviewflag(gcbh); end  DeleteFcn=if exist('delete_tlblock','file')==2,delete_tlblock(gcbh);end  NameChangeFcn=if exist('rename_tlblock','file')==2,rename_tlblock(gcbh);end  OpenFcn=if exist('tl_open_blockdlg','file')==2,tl_open_blockdlg(gcbh);else,open_system(gcbh,'parameter');end
      mask Help: eval(['if exist(''tl_online_help'',''file'') == 2, tl_online_help(''Topic'',''TL_Merge''),else, web([''jar:file:///'',matlabroot,''/help/toolbox/simulink/help.jar!/slref/' lower(get_param(gcbh,'Blocktype')) '.html''], ''-helpbrowser''),end'])
      mask Display: plot([-0.05, 1.05, NaN, -0.05, 1.05],[.01, .01, NaN, .99, .99])
  bStartOfDiagRequest_PRO : Logic  AllPortsSameDT=off  OutDataTypeStr=boolean  mask(TL_LogicalOperator){data={'output',{'name','$B'},'date',735626.4046887384}}
      settings: DeleteFcn=if exist('delete_tlblock','file')==2,delete_tlblock(gcbh);end  NameChangeFcn=if exist('rename_tlblock','file')==2,rename_tlblock(gcbh);end  OpenFcn=if exist('tl_open_blockdlg','file')==2,tl_open_blockdlg(gcbh);else,open_system(gcbh,'parameter');end
      mask Help: eval(['if exist(''tl_online_help'',''file'') == 2, tl_online_help(''Topic'',''TL_LogicalOperator''),else, web([''jar:file:///'',matlabroot,''/help/toolbox/simulink/help.jar!/slref/' lower(get_param(gcbh,'Blocktype')) '.html''], ''-helpbrowser''),end'])
      mask Display: plot([-0.05, 1.05, NaN, -0.05, 1.05],[.01, .01, NaN, .99, .99])
  bPreActivationFlag_PRO : Outport  InitialOutput=[0]
  wires:
  [u8RequestedCycle] -> bDiagRequest_PRO/1
  [u8ProdCycleId] -> bDiagRequest_PRO/2
  [u8ProdCycleId] -> bNoDiagRequest_PRO/2
  [u8PreviousRequestedCycle] -> bNoDiagRequest_PRO/1
  bNoDiagRequest_PRO/1 -> bStartOfDiagRequest_PRO/1
  bDiagRequest_PRO/1 -> bStartOfDiagRequest_PRO/2
  bStartOfDiagRequest_PRO/1 -> Set activation/1(In1), If/1
  If/1 -> Set activation/Action
  If/2 -> Clear activation/Action
  If/3 -> Keep activation/Action
  Set activation/1(Out1) -> bPreActivation_PRO/1
  Clear activation/1(Out1) -> bPreActivation_PRO/2
  Keep activation/1(Out1) -> bPreActivation_PRO/3
  bPreActivation_PRO/1 -> bPreActivationFlag_PRO/1
  bAcquitePreActivation_PRO/1 -> Clear activation/1(In1)
  [u8RequestedCycle] -> bNoMoreDiagRequest_PRO/1
  [u8ProdCycleId] -> bNoMoreDiagRequest_PRO/2
  bNoMoreDiagRequest_PRO/1 -> bClearActivation_PRO/2
  bClearActivation_PRO/1 -> If/2, bAcquitePreActivation_PRO/1
  [bEndOfExecutedCycle] -> bClearActivation_PRO/1
  u8CycleNumber/1 -> [u8CycleNumber]
  u8DiagRequestedCycle/1 -> [u8RequestedCycle]
  u8PreviousExecutedCycle/1 -> [u8PreviousExecutedCycle]
  u8PreviousRequestedCycle/1 -> [u8PreviousRequestedCycle]
  [u8ProdCycleId] -> bDiagRequest_BSR7/2
  bDiagRequest_BSR7/1 -> bDecideToAcquiteDiagRequestFromDIA/1
  [u8RequestedCycle] -> bDiagRequest_BSR6/1
  [u8ProdCycleId] -> bDiagRequest_BSR6/2
  [u8PreviousRequestedCycle] -> bDiagRequest_BSR7/1
  bDiagRequest_BSR6/1 -> bDecideToAcquiteDiagRequestFromDIA/2
  [bEndOfExecutedCycle] -> bDecideToAcquiteDiagRequestFromDIA/3
  bDecideToAcquiteDiagRequestFromDIA/1 -> If1/1
  If1/1 -> Acquite Diag Request From DIA/Action
  bDiagRequest_BSR1/1 -> bEndOfExecutedCycle_PRO/1
  bDiagRequest_BSR2/1 -> bEndOfExecutedCycle_PRO/2
  [u8PreviousExecutedCycle] -> bDiagRequest_BSR1/1
  [u8ProdCycleId] -> bDiagRequest_BSR2/2
  [u8ProdCycleId] -> bDiagRequest_BSR1/2
  [u8CycleNumber] -> bDiagRequest_BSR2/1
  bEndOfExecutedCycle_PRO/1 -> [bEndOfExecutedCycle]
  u8ProdCycleId/1 -> [u8ProdCycleId]
  bMemoryPreActivation/1 -> [bMemoryPreActivation]
  [bMemoryPreActivation] -> Keep activation/1(In1)

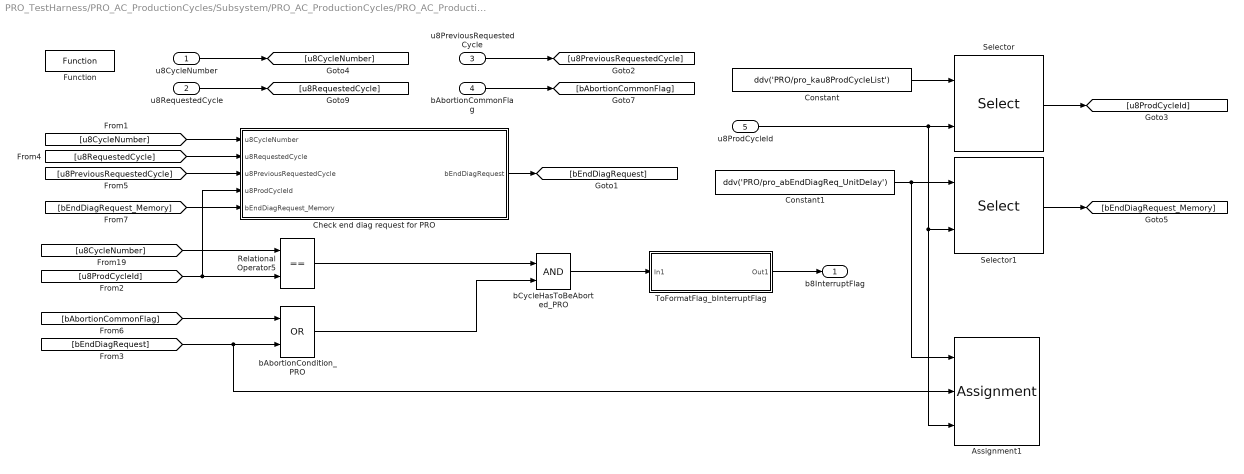
== system PRO_TestHarness/PRO_AC_ProductionCycles/Subsystem/PRO_AC_ProductionCycles/PRO_AC_ProductionCycles/PRO_runProductionCycles/PRO enabled/FctTrigAbortCycle_AllPRO/For Iterator Subsystem/Algo PRO/FctAbort_PRO ==
  u8CycleNumber : Inport  PortDimensions=1
  u8RequestedCycle : Inport  Port=2  OutDataTypeStr=uint8  PortDimensions=1
  u8PreviousRequestedCycle : Inport  Port=3  OutDataTypeStr=uint8  PortDimensions=1
  bAbortionCommonFlag : Inport  Port=4
  u8ProdCycleId : Inport  Port=5  PortDimensions=1
  Assignment1 : Assignment  IndexMode=Zero-based  IndexOptions=Index vector (port)  Indices=1  OutputSizes=1  mask(TL_Assignment){data={'output',{'variable','PRO/pro_abEndDiagReq_UnitDelay','inheritscaling',0},'date',736182.67238098383}}
      settings: CopyFcn=if exist('tl_reset_reviewflag') == 2, tl_reset_reviewflag(gcbh); end  DeleteFcn=if exist('delete_tlblock','file')==2,delete_tlblock(gcbh);end  NameChangeFcn=if exist('rename_tlblock','file')==2,rename_tlblock(gcbh);end  OpenFcn=if exist('tl_open_blockdlg','file')==2,tl_open_blockdlg(gcbh);else,open_system(gcbh,'parameter');end
      mask Help: eval(['if exist(''tl_online_help'',''file'') == 2, tl_online_help(''Topic'',''TL_Assignment''),else, web([''jar:file:///'',matlabroot,''/help/toolbox/simulink/help.jar!/slref/' lower(get_param(gcbh,'Blocktype')) '.html''], ''-helpbrowser''),end'])
      mask Display: plot([-0.05, 1.05, NaN, -0.05, 1.05],[.01, .01, NaN, .99, .99])
  Check end diag request for PRO : Subsystem
  Constant : Constant  Value=ddv('PRO/pro_kau8ProdCycleList')  mask(TL_Constant){data={'output',{'variable','PRO/pro_kau8ProdCycleList'},'date',736182.43287164357}}
      settings: CopyFcn=if exist('tl_reset_reviewflag') == 2, tl_reset_reviewflag(gcbh); end  DeleteFcn=if exist('delete_tlblock','file')==2,delete_tlblock(gcbh);end  NameChangeFcn=if exist('rename_tlblock','file')==2,rename_tlblock(gcbh);end  OpenFcn=if exist('tl_open_blockdlg','file')==2,tl_open_blockdlg(gcbh);else,open_system(gcbh,'parameter');end
      mask Help: eval(['if exist(''tl_online_help'',''file'') == 2, tl_online_help(''Topic'',''TL_Constant''),else, web([''jar:file:///'',matlabroot,''/help/toolbox/simulink/help.jar!/slref/' lower(get_param(gcbh,'Blocktype')) '.html''], ''-helpbrowser''),end'])
      mask Display: plot([-0.05, 1.05, NaN, -0.05, 1.05],[.01, .01, NaN, .99, .99])
  Constant1 : Constant  Value=ddv('PRO/pro_abEndDiagReq_UnitDelay')  OutDataTypeStr=boolean  mask(TL_Constant){data={'output',{'variable','PRO/pro_abEndDiagReq_UnitDelay'},'date',736182.66698633099}}
      settings: CopyFcn=if exist('tl_reset_reviewflag') == 2, tl_reset_reviewflag(gcbh); end  DeleteFcn=if exist('delete_tlblock','file')==2,delete_tlblock(gcbh);end  NameChangeFcn=if exist('rename_tlblock','file')==2,rename_tlblock(gcbh);end  OpenFcn=if exist('tl_open_blockdlg','file')==2,tl_open_blockdlg(gcbh);else,open_system(gcbh,'parameter');end
      mask Help: eval(['if exist(''tl_online_help'',''file'') == 2, tl_online_help(''Topic'',''TL_Constant''),else, web([''jar:file:///'',matlabroot,''/help/toolbox/simulink/help.jar!/slref/' lower(get_param(gcbh,'Blocktype')) '.html''], ''-helpbrowser''),end'])
      mask Display: plot([-0.05, 1.05, NaN, -0.05, 1.05],[.01, .01, NaN, .99, .99])
  Function : tllib/Function  data={'stepfunctionname','AbortPRO','stepfunctionclass','STATIC_FCN_ASR4','codecomment',['This function is in charge of' char(10) 'providing the following outputs:' char(10) '' char(10) '- Abortion flag for PRO1 cycle' char(10) '' char(10) 'according to the inputs:' char(10) '' char(10) '- executed cycle number' char(10) '- consistent cycle requested by diagnostic' char(10) '- previous (10 ms before) consistent cycle requested by diagnostic' char(10) '- common PRO abortion flag'],'module','PRO_AC_ProductionCycles','date',736463.55393709487}  displayString=FUNCTION
  Relational Operator5 : RelationalOperator  Operator===  OutDataTypeStr=boolean  mask(TL_RelationalOperator){data={'date',734825.61632244207}}
      settings: DeleteFcn=if exist('delete_tlblock','file')==2,delete_tlblock(gcbh);end  NameChangeFcn=if exist('rename_tlblock','file')==2,rename_tlblock(gcbh);end  OpenFcn=if exist('tl_open_blockdlg','file')==2,tl_open_blockdlg(gcbh);else,open_system(gcbh,'parameter');end
      mask Help: eval(['if exist(''tl_online_help'',''file'') == 2, tl_online_help(''Topic'',''TL_RelationalOperator''),else, web([''jar:file:///'',matlabroot,''/help/toolbox/simulink/help.jar!/slref/' lower(get_param(gcbh,'Blocktype')) '.html''], ''-helpbrowser''),end'])
      mask Display: plot([-0.05, 1.05, NaN, -0.05, 1.05],[.01, .01, NaN, .99, .99])
  Selector : Selector  IndexMode=Zero-based  InputPortWidth=2  IndexOptions=Index vector (port)  Indices=[1 3]  OutputSizes=1
  Selector1 : Selector  IndexMode=Zero-based  InputPortWidth=2  IndexOptions=Index vector (port)  Indices=[1 3]  OutputSizes=1
  ToFormatFlag_bInterruptFlag : Subsystem
  bAbortionCondition_PRO : Logic  Operator=OR  AllPortsSameDT=off  OutDataTypeStr=boolean  mask(TL_LogicalOperator){data={'output',{'name','$B'},'date',735643.4519548032}}
      settings: DeleteFcn=if exist('delete_tlblock','file')==2,delete_tlblock(gcbh);end  NameChangeFcn=if exist('rename_tlblock','file')==2,rename_tlblock(gcbh);end  OpenFcn=if exist('tl_open_blockdlg','file')==2,tl_open_blockdlg(gcbh);else,open_system(gcbh,'parameter');end
      mask Help: eval(['if exist(''tl_online_help'',''file'') == 2, tl_online_help(''Topic'',''TL_LogicalOperator''),else, web([''jar:file:///'',matlabroot,''/help/toolbox/simulink/help.jar!/slref/' lower(get_param(gcbh,'Blocktype')) '.html''], ''-helpbrowser''),end'])
      mask Display: plot([-0.05, 1.05, NaN, -0.05, 1.05],[.01, .01, NaN, .99, .99])
  bCycleHasToBeAborted_PRO : Logic  AllPortsSameDT=off  OutDataTypeStr=boolean  mask(TL_LogicalOperator){data={'output',{'name','$B'},'date',735605.60308376153}}
      settings: DeleteFcn=if exist('delete_tlblock','file')==2,delete_tlblock(gcbh);end  NameChangeFcn=if exist('rename_tlblock','file')==2,rename_tlblock(gcbh);end  OpenFcn=if exist('tl_open_blockdlg','file')==2,tl_open_blockdlg(gcbh);else,open_system(gcbh,'parameter');end
      mask Help: eval(['if exist(''tl_online_help'',''file'') == 2, tl_online_help(''Topic'',''TL_LogicalOperator''),else, web([''jar:file:///'',matlabroot,''/help/toolbox/simulink/help.jar!/slref/' lower(get_param(gcbh,'Blocktype')) '.html''], ''-helpbrowser''),end'])
      mask Display: plot([-0.05, 1.05, NaN, -0.05, 1.05],[.01, .01, NaN, .99, .99])
  b8InterruptFlag : Outport  PortDimensions=1
  wires:
  u8CycleNumber/1 -> [u8CycleNumber]
  [u8CycleNumber] -> Relational Operator5/1
  [u8ProdCycleId] -> Relational Operator5/2, Check end diag request for PRO/4(u8ProdCycleId)
  bCycleHasToBeAborted_PRO/1 -> ToFormatFlag_bInterruptFlag/1(In1)
  bAbortionCondition_PRO/1 -> bCycleHasToBeAborted_PRO/2
  Relational Operator5/1 -> bCycleHasToBeAborted_PRO/1
  bAbortionCommonFlag/1 -> [bAbortionCommonFlag]
  [bEndDiagRequest] -> Assignment1/2, bAbortionCondition_PRO/2
  ToFormatFlag_bInterruptFlag/1(Out1) -> b8InterruptFlag/1
  u8RequestedCycle/1 -> [u8RequestedCycle]
  [bAbortionCommonFlag] -> bAbortionCondition_PRO/1
  u8PreviousRequestedCycle/1 -> [u8PreviousRequestedCycle]
  [u8CycleNumber] -> Check end diag request for PRO/1(u8CycleNumber)
  [u8RequestedCycle] -> Check end diag request for PRO/2(u8RequestedCycle)
  [u8PreviousRequestedCycle] -> Check end diag request for PRO/3(u8PreviousRequestedCycle)
  Check end diag request for PRO/1(bEndDiagRequest) -> [bEndDiagRequest]
  Constant/1 -> Selector/1
  u8ProdCycleId/1 -> Assignment1/3, Selector1/2, Selector/2
  Selector/1 -> [u8ProdCycleId]
  Selector1/1 -> [bEndDiagRequest_Memory]
  Constant1/1 -> Assignment1/1, Selector1/1
  [bEndDiagRequest_Memory] -> Check end diag request for PRO/5(bEndDiagRequest_Memory)
